simulink model "table"  (R2023a)
settings: Solver=VariableStepAuto  StartTime=0.0  StopTime=10.0  RelTol=1e-3
values from neighbouring files (symbols this model uses):
  ts = struct('orig_30kph', ts_orig_30kph, 'gen_30kph', ts_gen_30kph, 'orig_40kph', ts_orig_40kph, 'gen_40kph', ts_gen_40kph, 'orig_50kph', ts_orig_50kph, 'gen_50kph', ts_gen_50kph, 'orig_60kph', ts_orig_60kph, 'gen_60kph', ts_gen_60kph,'orig_70kph', ts_orig_70kph, 'gen_70kph', ts_gen_70kph, 'orig_80kph', ts_orig_80kph, 'gen_80kph', ts_gen_80kph, 'orig_90kph', ts_orig_90kph, 'gen_90kph', ts_gen_90kph)    [data_to_mat.m]
settings Model: Creator=safder.1  LastModifiedBy=kazishb
settings OptimizationCC: ReuseModelBlockBuffer=off

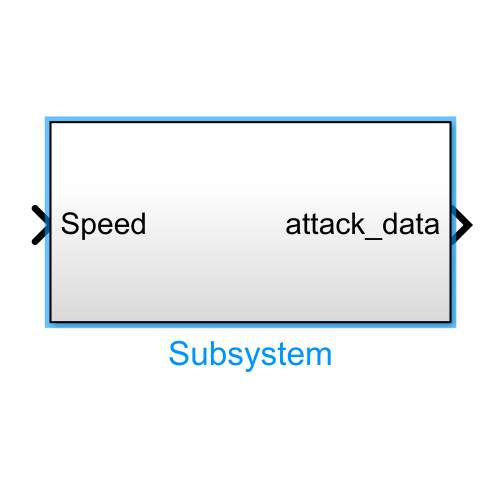
[thumbnail: Simulink's stored preview of the top-level diagram]
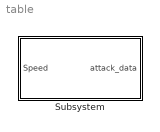
== system table ==
  Subsystem : Subsystem

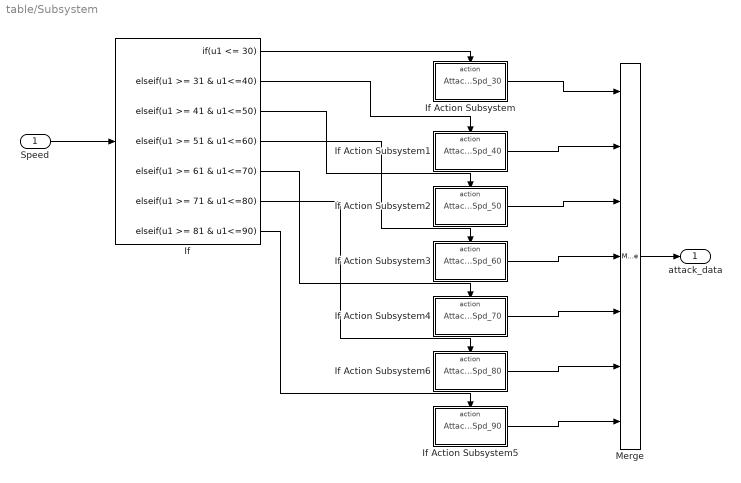
== system table/Subsystem ==
  Speed : Inport
  If : If  IfExpression=u1 <= 30  ElseIfExpressions=u1 >= 31 & u1<=40,u1 >= 41 & u1<=50,u1 >= 51 & u1<=60,u1 >= 61 & u1<=70,u1 >= 71 & u1<=80,u1 >= 81 & u1<=90  ShowElse=off
  If Action Subsystem : Subsystem  TreatAsAtomicUnit=on
  If Action Subsystem1 : Subsystem  TreatAsAtomicUnit=on
  If Action Subsystem2 : Subsystem  TreatAsAtomicUnit=on
  If Action Subsystem3 : Subsystem  TreatAsAtomicUnit=on
  If Action Subsystem4 : Subsystem  TreatAsAtomicUnit=on
  If Action Subsystem5 : Subsystem  TreatAsAtomicUnit=on
  If Action Subsystem6 : Subsystem  TreatAsAtomicUnit=on
  Merge : Merge  Inputs=7
  attack_data : Outport
  wires:
  If/5 -> If Action Subsystem4/Action
  If/4 -> If Action Subsystem3/Action
  If Action Subsystem1/1(AttachSpd_40) -> Merge/2
  If Action Subsystem3/1(AttachSpd_60) -> Merge/4
  If Action Subsystem/1(AttachSpd_30) -> Merge/1
  If Action Subsystem2/1(AttachSpd_50) -> Merge/3
  If/1 -> If Action Subsystem/Action
  If Action Subsystem4/1(AttachSpd_70) -> Merge/5
  If Action Subsystem6/1(AttachSpd_80) -> Merge/6
  If Action Subsystem5/1(AttachSpd_90) -> Merge/7
  If/6 -> If Action Subsystem6/Action
  Speed/1 -> If/1
  Merge/1 -> attack_data/1
  If/2 -> If Action Subsystem1/Action
  If/3 -> If Action Subsystem2/Action
  If/7 -> If Action Subsystem5/Action

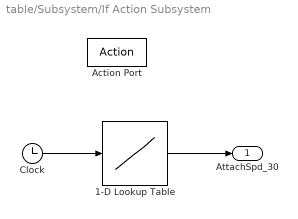
== system table/Subsystem/If Action Subsystem ==
  Action Port : ActionPort  ActionPortLabel=if(u1 <= 30)
  1-D Lookup Table : Lookup_n-D  NumberOfTableDimensions=1  BreakpointsForDimension1=ts.orig_30kph.Time  Table=ts.gen_30kph.Data  InternalRulePriority=Speed  RndMeth=Simplest
  Clock : Clock
  AttachSpd_30 : Outport
  wires:
  Clock/1 -> 1-D Lookup Table/1
  1-D Lookup Table/1 -> AttachSpd_30/1

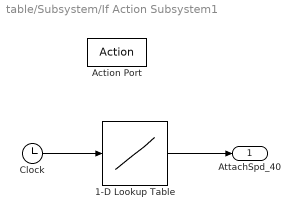
== system table/Subsystem/If Action Subsystem1 ==
  Action Port : ActionPort  ActionPortLabel=elseif(u1 >= 31 & u1<=40)
  1-D Lookup Table : Lookup_n-D  NumberOfTableDimensions=1  BreakpointsForDimension1=ts.orig_40kph.Time  Table=ts.gen_40kph.Data  InternalRulePriority=Speed  RndMeth=Simplest
  Clock : Clock
  AttachSpd_40 : Outport
  wires:
  Clock/1 -> 1-D Lookup Table/1
  1-D Lookup Table/1 -> AttachSpd_40/1

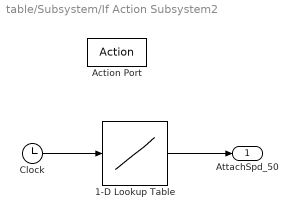
== system table/Subsystem/If Action Subsystem2 ==
  Action Port : ActionPort  ActionPortLabel=elseif(u1 >= 41 & u1<=50)
  1-D Lookup Table : Lookup_n-D  NumberOfTableDimensions=1  BreakpointsForDimension1=ts.orig_50kph.Time  Table=ts.gen_50kph.Data  InternalRulePriority=Speed  RndMeth=Simplest
  Clock : Clock
  AttachSpd_50 : Outport
  wires:
  Clock/1 -> 1-D Lookup Table/1
  1-D Lookup Table/1 -> AttachSpd_50/1

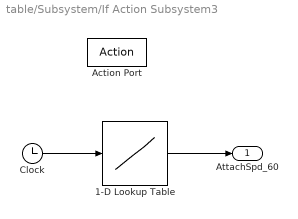
== system table/Subsystem/If Action Subsystem3 ==
  Action Port : ActionPort  ActionPortLabel=elseif(u1 >= 51 & u1<=60)
  1-D Lookup Table : Lookup_n-D  NumberOfTableDimensions=1  BreakpointsForDimension1=ts.orig_60kph.Time  Table=ts.gen_60kph.Data  InternalRulePriority=Speed  RndMeth=Simplest
  Clock : Clock
  AttachSpd_60 : Outport
  wires:
  Clock/1 -> 1-D Lookup Table/1
  1-D Lookup Table/1 -> AttachSpd_60/1

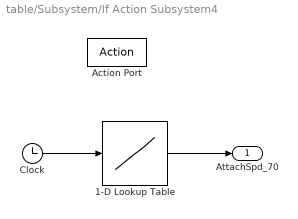
== system table/Subsystem/If Action Subsystem4 ==
  Action Port : ActionPort  ActionPortLabel=elseif(u1 >= 61 & u1<=70)
  1-D Lookup Table : Lookup_n-D  NumberOfTableDimensions=1  BreakpointsForDimension1=ts.orig_70kph.Time  Table=ts.gen_70kph.Data  InternalRulePriority=Speed  RndMeth=Simplest
  Clock : Clock
  AttachSpd_70 : Outport
  wires:
  Clock/1 -> 1-D Lookup Table/1
  1-D Lookup Table/1 -> AttachSpd_70/1

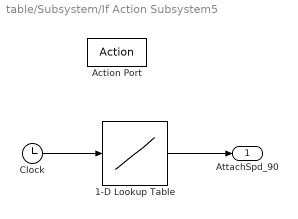
== system table/Subsystem/If Action Subsystem5 ==
  Action Port : ActionPort  ActionPortLabel=elseif(u1 >= 81 & u1<=90)
  1-D Lookup Table : Lookup_n-D  NumberOfTableDimensions=1  BreakpointsForDimension1=ts.orig_90kph.Time  Table=ts.gen_90kph.Data  InternalRulePriority=Speed  RndMeth=Simplest
  Clock : Clock
  AttachSpd_90 : Outport
  wires:
  Clock/1 -> 1-D Lookup Table/1
  1-D Lookup Table/1 -> AttachSpd_90/1

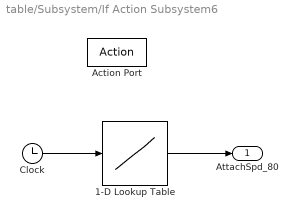
== system table/Subsystem/If Action Subsystem6 ==
  Action Port : ActionPort  ActionPortLabel=elseif(u1 >= 71 & u1<=80)
  1-D Lookup Table : Lookup_n-D  NumberOfTableDimensions=1  BreakpointsForDimension1=ts.orig_80kph.Time  Table=ts.gen_80kph.Data  InternalRulePriority=Speed  RndMeth=Simplest
  Clock : Clock
  AttachSpd_80 : Outport
  wires:
  Clock/1 -> 1-D Lookup Table/1
  1-D Lookup Table/1 -> AttachSpd_80/1
